simulink model "testat_2_b2"  (R2016a)
settings: Solver=VariableStepAuto  StartTime=0.0  StopTime=20  MaxStep=0.01  RelTol=1e-3
values from neighbouring files (symbols this model uses):
  c = 1.2    [testat2_a1.m]
  D = 1.2    [testat2_a1.m]
  m = 4.5    [testat2_a1.m]
  y0 = 1    [testat2_a1.m]
settings Model: Creator=bachman0  LastModifiedBy=bachman0

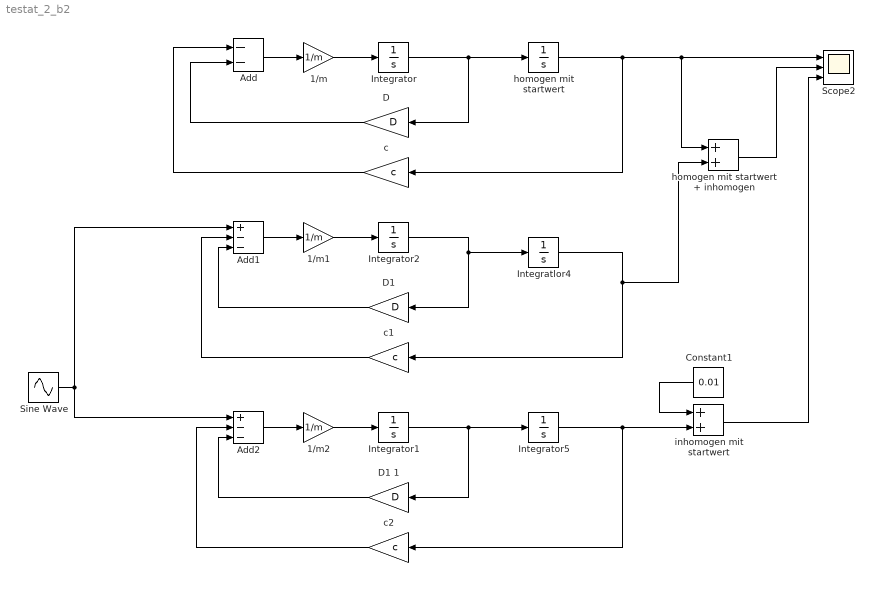
== system testat_2_b2 ==
  1/m : Gain  Gain=1/m
  1/m1 : Gain  Gain=1/m
  1/m2 : Gain  Gain=1/m
  Add : Sum  Inputs=--
  Add1 : Sum  Inputs=+--
  Add2 : Sum  Inputs=+--
  Constant1 : Constant  Value=0.01
  "D\t" : Gain  Gain=D
  "D1\t" : Gain  Gain=D
  D1	1 : Gain  Gain=D
  Integratlor4 : Integrator
  Integrator : Integrator
  Integrator1 : Integrator
  Integrator2 : Integrator
  Integrator5 : Integrator  InitialCondition=y0
  Scope2 : Scope  NumInputPorts=3
  Sine Wave : Sin  Amplitude=10  Frequency=5  Phase=pi/2  SampleTime=0
  c : Gain  Gain=c
  c1 : Gain  Gain=c
  c2 : Gain  Gain=c
  homogen mit startwert : Integrator  InitialCondition=y0
  homogen mit startwert + inhomogen : Sum
  inhomogen mit startwert : Sum
  wires:
  Integrator/1 -> "D\t"/1, homogen mit startwert/1
  homogen mit startwert/1 -> c/1, homogen mit startwert + inhomogen/1, Scope2/1
  "D\t"/1 -> Add/2
  c/1 -> Add/1
  Integrator2/1 -> "D1\t"/1, Integratlor4/1
  Integratlor4/1 -> c1/1, homogen mit startwert + inhomogen/2
  "D1\t"/1 -> Add1/3
  c1/1 -> Add1/2
  Add/1 -> 1/m/1
  Add1/1 -> 1/m1/1
  Integrator1/1 -> D1	1/1, Integrator5/1
  Integrator5/1 -> inhomogen mit startwert/2, c2/1
  D1	1/1 -> Add2/3
  c2/1 -> Add2/2
  Add2/1 -> 1/m2/1
  Constant1/1 -> inhomogen mit startwert/1
  homogen mit startwert + inhomogen/1 -> Scope2/2
  inhomogen mit startwert/1 -> Scope2/3
  1/m2/1 -> Integrator1/1
  1/m1/1 -> Integrator2/1
  1/m/1 -> Integrator/1
  Sine Wave/1 -> Add2/1, Add1/1
